simulink library "ETRobocon2013Plant_lib"  (R2013b)
settings: Solver=ode45  StartTime=0.0  StopTime=10.0  RelTol=1e-3
undefined symbols (not defined in the file): rWheel
libraries: fl_lib x5
settings Model: Creator=scastro  LastModifiedBy=scastro

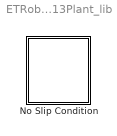
== system ETRobocon2013Plant_lib ==
  No Slip Condition : Subsystem
      settings: MinAlgLoopOccurrences=on

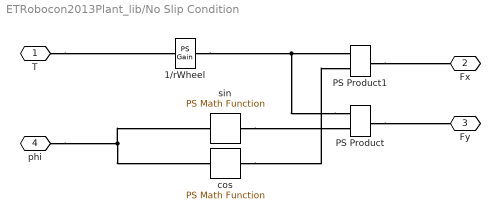
== system ETRobocon2013Plant_lib/No Slip Condition ==
  1/rWheel : fl_lib/Physical Signals/Functions/PS Gain  gain=1/rWheel  LocalVarLogging=[]
  PS Product : fl_lib/Physical Signals/Functions/PS Product  LocalVarLogging=[]
  PS Product1 : fl_lib/Physical Signals/Functions/PS Product  LocalVarLogging=[]
  cos : fl_lib/Physical Signals/Functions/PS Math Function  fcn_choice=2  LocalVarLogging=[]
  sin : fl_lib/Physical Signals/Functions/PS Math Function  fcn_choice=1  LocalVarLogging=[]
  T : PMIOPort  Port=1  Side=Left
  Fx : PMIOPort  Port=2  Side=Right
  Fy : PMIOPort  Port=3  Side=Right
  phi : PMIOPort  Port=4  Side=Left
  connections:
  PS Product/RConn1 -- Fy/RConn1
  PS Product1/RConn1 -- Fx/RConn1
  T/RConn1 -- 1/rWheel/LConn1
  PS Product/LConn1 -- PS Product1/LConn1 -- 1/rWheel/RConn1
  sin/RConn1 -- PS Product/LConn2
  cos/RConn1 -- PS Product1/LConn2
  phi/RConn1 -- sin/LConn1 -- cos/LConn1
